simulink model "Dynamic"  (R2015a)
settings: Solver=ode5  StartTime=0.0  StopTime=15  FixedStep=0.001  RelTol=1e-3
values from neighbouring files (symbols this model uses):
  a = 0.15    [Init.m]    (also in lyapu.m; plotKinematic.m = 0.13)
  a_e = (1 + err_a)*a    (= 0.15)    [Init.m]
  d = 0.05    [Init.m]    (also in plotKinematic.m = 0.1)
  Kd = 10    [Init.m]
  Kp = 25    [Init.m]
  r = 0.1    [Init.m]    (also in plotKinematic.m)
  R = 2    [Init.m]
  r_e = (1 + err_r)*r    (= 0.1)    [Init.m]
  theta0 = pi    (= 3.14159265359)    [Init.m]
  wd = 0.5    [Init.m]
  x0 = 2.3    [Init.m]
  y0 = 0    [Init.m]
settings Model: Creator=tgvo  LastModifiedBy=tgvo
settings DataIOCC: LimitDataPoints=off

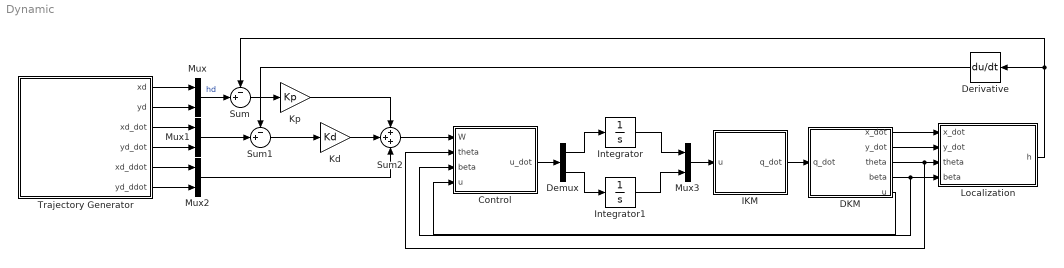
== system Dynamic ==
  Control : Subsystem  mask{a=a, d=d}
  DKM : Subsystem  mask{a=a, r=r, d=d}
  Demux : Demux  Outputs=2
  Derivative : Derivative
  IKM : Subsystem  mask{L_e=a_e, r_e=r_e}
      mask prompts: L_e "Estimated distance b/w steerable wheel and Om"; r_e "Estimated wheel radius"
  Integrator : Integrator
  Integrator1 : Integrator
  Kd : Gain  Gain=Kd
  Kp : Gain  Gain=Kp
  Localization : Subsystem  mask{a=a, d=d, x0=x0, y0=y0}
      mask prompts: a "Value of a"; d "Value of d"; x0 "Initial value of x"; y0 "Initial value of y"
  Mux{,1..3} (4 alike) : Mux  Inputs=2
  Sum : Sum  Inputs=-+|
  Sum1 : Sum  Inputs=-+|
  Sum2 : Sum  Inputs=+++
  Trajectory Generator : Subsystem  mask{R=R, wd=wd}
      mask prompts: R "Circular Radius"; wd "Desired Angular Velocity"
  wires:
  Trajectory Generator/1(xd) -> Mux/1
  Trajectory Generator/6(yd_ddot) -> Mux2/2
  Mux1/1 -> Sum1/2
  Sum1/1 -> Kd/1
  Kd/1 -> Sum2/2
  Kp/1 -> Sum2/1
  Mux2/1 -> Sum2/3
  Sum2/1 -> Control/1(W)
  Control/1(u_dot) -> Demux/1
  Demux/1 -> Integrator/1
  Demux/2 -> Integrator1/1
  Integrator/1 -> Mux3/1
  Integrator1/1 -> Mux3/2
  Mux3/1 -> IKM/1(u)
  IKM/1(q_dot) -> DKM/1(q_dot)
  DKM/5(u) -> Control/4(u)
  Localization/1(h) -> Sum/1, Derivative/1
  Derivative/1 -> Sum1/1
  Mux/1 -> Sum/2  "hd"
  Sum/1 -> Kp/1
  DKM/4(beta) -> Control/3(beta), Localization/4(beta)
  DKM/3(theta) -> Control/2(theta), Localization/3(theta)
  DKM/2(y_dot) -> Localization/2(y_dot)
  DKM/1(x_dot) -> Localization/1(x_dot)
  Trajectory Generator/2(yd) -> Mux/2
  Trajectory Generator/3(xd_dot) -> Mux1/1
  Trajectory Generator/4(yd_dot) -> Mux1/2
  Trajectory Generator/5(xd_ddot) -> Mux2/1

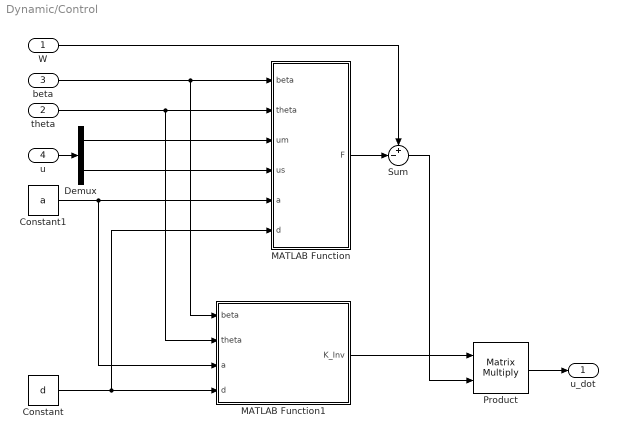
== system Dynamic/Control ==
  W : Inport
  theta : Inport  Port=2
  beta : Inport  Port=3
  u : Inport  Port=4
  Constant : Constant  Value=d
  Constant1 : Constant  Value=a
  Demux : Demux  Outputs=2
  MATLAB Function : MATLAB Function  TreatAsAtomicUnit=on
  MATLAB Function1 : MATLAB Function  TreatAsAtomicUnit=on
  Product : Product  Multiplication=Matrix(*)
  Sum : Sum  Inputs=+-|
  u_dot : Outport
  wires:
  Constant/1 -> MATLAB Function/6(d), MATLAB Function1/4(d)
  Constant1/1 -> MATLAB Function1/3(a), MATLAB Function/5(a)
  theta/1 -> MATLAB Function1/2(theta), MATLAB Function/2(theta)
  beta/1 -> MATLAB Function1/1(beta), MATLAB Function/1(beta)
  MATLAB Function/1(F) -> Sum/2
  W/1 -> Sum/1
  MATLAB Function1/1(K_Inv) -> Product/1
  Sum/1 -> Product/2
  Product/1 -> u_dot/1
  u/1 -> Demux/1
  Demux/1 -> MATLAB Function/3(um)
  Demux/2 -> MATLAB Function/4(us)

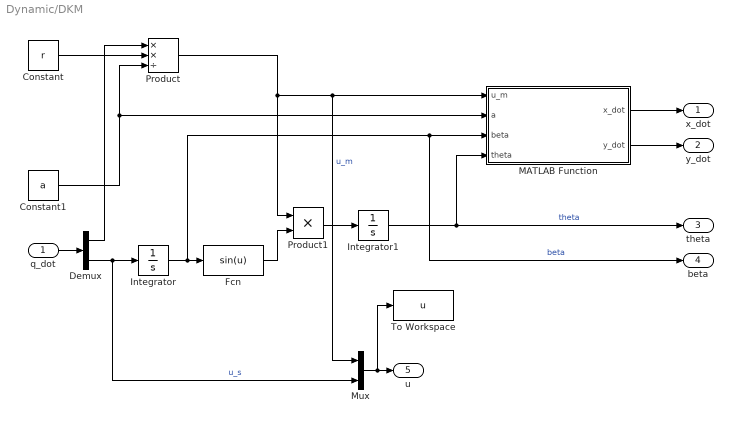
== system Dynamic/DKM ==
  q_dot : Inport
  Constant : Constant  Value=r
  Constant1 : Constant  Value=a
  Demux : Demux  Outputs=2
  Fcn : Fcn  Expr=sin(u)
  Integrator : Integrator
  Integrator1 : Integrator  InitialCondition=theta0
  MATLAB Function : MATLAB Function  TreatAsAtomicUnit=on
  Mux : Mux  Inputs=2
  Product : Product  Inputs=**/
  Product1 : Product
  To Workspace : ToWorkspace  VariableName=u  SampleTime=-1
  x_dot : Outport
  y_dot : Outport  Port=2
  theta : Outport  Port=3
  beta : Outport  Port=4
  u : Outport  Port=5
  wires:
  Constant/1 -> Product/2
  Demux/1 -> Product/1
  Integrator/1 -> beta/1, MATLAB Function/3(beta), Fcn/1  "beta"
  Fcn/1 -> Product1/2
  Product/1 -> Mux/1, MATLAB Function/1(u_m), Product1/1  "u_m"
  Product1/1 -> Integrator1/1
  q_dot/1 -> Demux/1
  Demux/2 -> Mux/2, Integrator/1  "u_s"
  Constant1/1 -> Product/3, MATLAB Function/2(a)
  Integrator1/1 -> theta/1, MATLAB Function/4(theta)  "theta"
  MATLAB Function/2(y_dot) -> y_dot/1
  Mux/1 -> To Workspace/1, u/1
  MATLAB Function/1(x_dot) -> x_dot/1

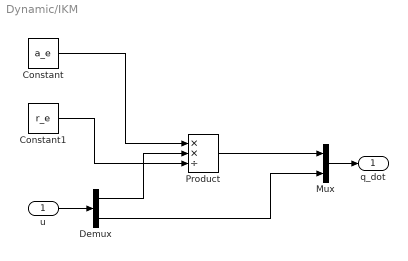
== system Dynamic/IKM ==
  u : Inport
  Constant : Constant  Value=a_e
  Constant1 : Constant  Value=r_e
  Demux : Demux  Outputs=2
  Mux : Mux  Inputs=2
  Product : Product  Inputs=**/
  q_dot : Outport
  wires:
  u/1 -> Demux/1
  Constant/1 -> Product/1
  Demux/1 -> Product/2
  Constant1/1 -> Product/3
  Mux/1 -> q_dot/1
  Product/1 -> Mux/1
  Demux/2 -> Mux/2

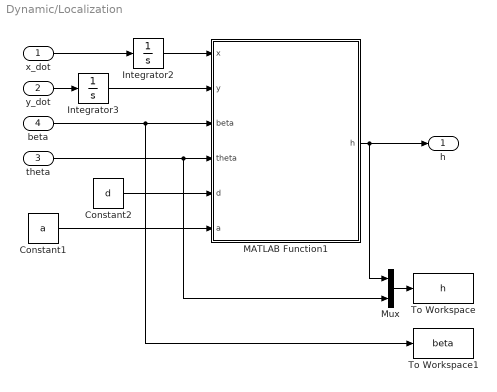
== system Dynamic/Localization ==
  x_dot : Inport
  y_dot : Inport  Port=2
  theta : Inport  Port=3
  beta : Inport  Port=4
  Constant1 : Constant  Value=a
  Constant2 : Constant  Value=d
  Integrator2 : Integrator  InitialCondition=x0
  Integrator3 : Integrator  InitialCondition=y0
  MATLAB Function1 : MATLAB Function  TreatAsAtomicUnit=on
  Mux : Mux  Inputs=2
  To Workspace : ToWorkspace  VariableName=h  SampleTime=-1
  To Workspace1 : ToWorkspace  VariableName=beta  SampleTime=-1
  h : Outport
  wires:
  Integrator2/1 -> MATLAB Function1/1(x)
  x_dot/1 -> Integrator2/1
  y_dot/1 -> Integrator3/1
  beta/1 -> To Workspace1/1, MATLAB Function1/3(beta)
  theta/1 -> Mux/2, MATLAB Function1/4(theta)
  MATLAB Function1/1(h) -> Mux/1, h/1
  Integrator3/1 -> MATLAB Function1/2(y)
  Constant2/1 -> MATLAB Function1/5(d)
  Constant1/1 -> MATLAB Function1/6(a)
  Mux/1 -> To Workspace/1

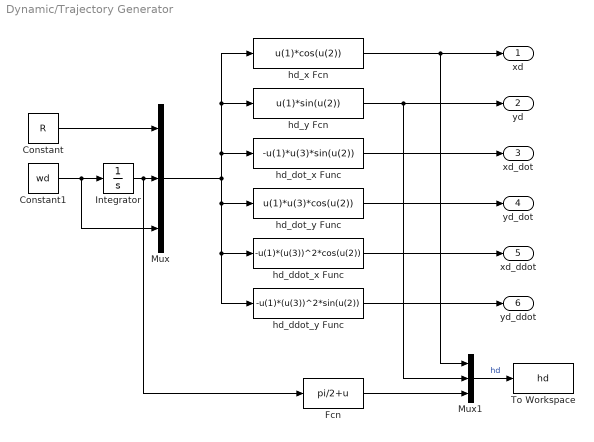
== system Dynamic/Trajectory Generator ==
  Constant : Constant  Value=R
  Constant1 : Constant  Value=wd
  Fcn : Fcn  Expr=pi/2+u
  Integrator : Integrator
  Mux : Mux  Inputs=3
  Mux1 : Mux  Inputs=3
  To Workspace : ToWorkspace  VariableName=hd  SampleTime=-1
  hd_ddot_x Func : Fcn  Expr=-u(1)*(u(3))^2*cos(u(2))
  hd_ddot_y Func : Fcn  Expr=-u(1)*(u(3))^2*sin(u(2))
  hd_dot_x Func : Fcn  Expr=-u(1)*u(3)*sin(u(2))
  hd_dot_y Func : Fcn  Expr=u(1)*u(3)*cos(u(2))
  hd_x Fcn : Fcn  Expr=u(1)*cos(u(2))
  hd_y Fcn : Fcn  Expr=u(1)*sin(u(2))
  xd : Outport
  yd : Outport  Port=2
  xd_dot : Outport  Port=3
  yd_dot : Outport  Port=4
  xd_ddot : Outport  Port=5
  yd_ddot : Outport  Port=6
  wires:
  hd_y Fcn/1 -> Mux1/2, yd/1
  hd_x Fcn/1 -> xd/1, Mux1/1
  Mux/1 -> hd_dot_x Func/1, hd_x Fcn/1, hd_y Fcn/1, hd_ddot_y Func/1, hd_ddot_x Func/1, hd_dot_y Func/1
  Constant1/1 -> Mux/3, Integrator/1
  Constant/1 -> Mux/1
  Mux1/1 -> To Workspace/1  "hd"
  Integrator/1 -> Fcn/1, Mux/2
  hd_dot_y Func/1 -> yd_dot/1
  hd_ddot_x Func/1 -> xd_ddot/1
  hd_dot_x Func/1 -> xd_dot/1
  hd_ddot_y Func/1 -> yd_ddot/1
  Fcn/1 -> Mux1/3

== matlab function Dynamic/Control/MATLAB Function1 ==
  data: beta input; K_Inv output; theta input; a input; d input
function K_Inv = Find_K_Inv(beta,theta,a,d)
%#codegen

K = [a*cos(beta+theta)-d*sin(beta+theta)*sin(beta), -d*sin(beta+theta);...
     a*sin(beta+theta)+d*cos(beta+theta)*sin(beta), d*cos(beta+theta)];
 K_Inv = inv(K);

== matlab function Dynamic/Control/MATLAB Function ==
  data: beta input; theta input; um input; us input; F output; a input; d input
function F = FxBlock(beta,theta,um,us,a,d)


F11 = -um^2*sin(beta)*(a*sin(beta+theta)+d*sin(beta)*cos(beta+theta))...
      -um*us*(a*sin(beta+theta)+2*d*sin(beta)*cos(beta+theta)+d*cos(beta)*sin(beta+theta))...
      -us^2*d*cos(beta+theta);
  
F21 = um^2*sin(beta)*(a*cos(beta+theta)-d*sin(beta)*sin(beta+theta))...
      +um*us*(a*cos(beta+theta)-2*d*sin(beta)*sin(beta+theta)+d*cos(beta)*cos(beta+theta))...
      -us^2*d*sin(beta+theta);

F = [F11;F21];

== matlab function Dynamic/DKM/MATLAB Function ==
  data: u_m input; x_dot output; a input; beta input; theta input; y_dot output
function [x_dot,y_dot] = Find_xy_dot(u_m,a,beta,theta)

x_dot = a*cos(beta)*cos(theta)*u_m;
y_dot = a*cos(beta)*sin(theta)*u_m;

== matlab function Dynamic/Localization/MATLAB Function1 ==
  data: x input; y input; beta input; theta input; d input; a input; h output
function h = Find_h(x,y,beta,theta,d,a)
%#codegen
z1 = x + a*cos(theta) + d*cos(theta+beta);
z2 = y + a*sin(theta) + d*sin(theta+beta);
h = [z1;z2];
